simulink model "systemControlHardware"  (R2022b)
settings: Solver=FixedStepAuto  StartTime=0.0  StopTime=.75  FixedStep=T  RelTol=1e-3
values from neighbouring files (symbols this model uses):
  alpha = 25    [dataControlHardware.mat]    (also in initControlHardware.m)
  alpha1 = 35.5    [dataControlHardware.mat]    (also in initControlHardware.m)
  G = 0.00157079632679    [dataControlHardware.mat]    (also in initControlHardware.m)
  H = 60    [dataControlHardware.mat]    (also in dataExperimentalOneVolt.mat = 1; dataExperimentalThreeVolt.mat = 3; dataExperimentalTwoVolt.mat = 2; initControlHardware.m)
  K = 0.2025    [dataControlHardware.mat]    (also in initControlHardware.m)
  Kf = 17.75    [dataControlHardware.mat]    (also in initControlHardware.m)
  T = 0.001    [dataControlHardware.mat]    (also in dataExperimentalOneVolt.mat; dataExperimentalThreeVolt.mat; dataExperimentalTwoVolt.mat; initControlHardware.m)
undefined symbols (not defined in the file or in its folder): Humusoft, MF634
libraries: sldrtlib x2
settings Model: SimulationMode=external  ExtModeTrigDuration=100000  Creator=oschnippering  LastModifiedBy=fwah
settings DataIOCC: ReturnWorkspaceOutputs=off
settings HardwareCC: ProdBitPerLong=64  ProdHWDeviceType=Intel->x86-64 (Linux 64)
settings ModelReferenceCC: EnableRefExpFcnMdlSchedulingChecks=on
settings RTWCC: Description=Simulink Desktop Real-Time  SystemTargetFile=sldrt.tlc  TemplateMakefile=sldrt.tmf  RTWCompilerOptimization=on
settings CodeAppCC: MaxIdLength=95
settings SimulinkDesktopRealTimeCC: TargetLibSuffix=_sldrt.a  TargetPreCompLibLocation=C:\Program Files\MATLAB\R2022b\toolbox\sldrt\lib\win64

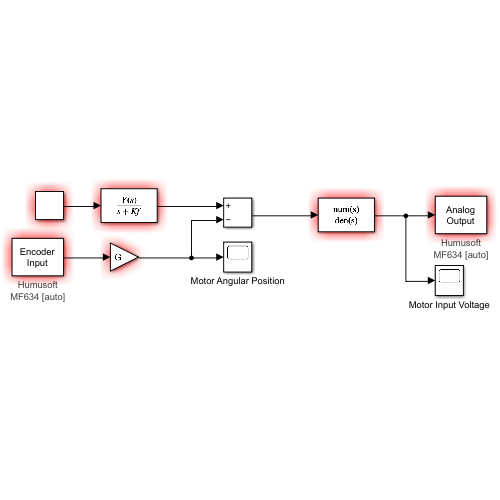
[thumbnail: Simulink's stored preview of the top-level diagram]
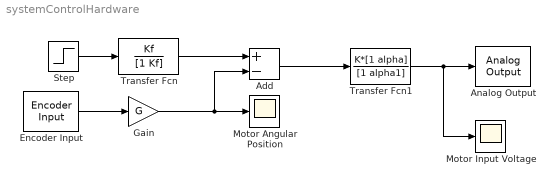
== system systemControlHardware ==
  Add : Sum  Inputs=+-
  Analog Output : sldrtlib/Analog Output  SampleTime=T  MaxMissedTicks=10  ShowMissedTicks=off  YieldWhenWaiting=off  DrvName=Humusoft/MF634  DrvAddress=4294967295  DrvOptions=0  Channels=1  RangeMode=1  VoltRange=1  InitialValue=0  FinalValue=0
      settings: AttributesFormatString=Humusoft\nMF634 [auto]
  Encoder Input : sldrtlib/Encoder Input  SampleTime=T  MaxMissedTicks=10  ShowMissedTicks=off  YieldWhenWaiting=off  DrvName=Humusoft/MF634  DrvAddress=4294967295  DrvOptions=0  Channels=1  QuadMode=3  IndexPulse=3  InputFilter=Inf  DataType=1
      settings: AttributesFormatString=Humusoft\nMF634 [auto]
  Gain : Gain  Gain=G
  Motor Angular Position : Scope
  Motor Input Voltage : Scope
  Step : Step  After=H  SampleTime=0
  Transfer Fcn : TransferFcn  Numerator=Kf  Denominator=[1 Kf]
  Transfer Fcn1 : TransferFcn  Numerator=K*[1 alpha]  Denominator=[1 alpha1]
  wires:
  Step/1 -> Transfer Fcn/1
  Transfer Fcn/1 -> Add/1
  Encoder Input/1 -> Gain/1
  Gain/1 -> Add/2, Motor Angular Position/1
  Add/1 -> Transfer Fcn1/1
  Transfer Fcn1/1 -> Motor Input Voltage/1, Analog Output/1
